simulink model "LQE_x"  (R2022a)
settings: Solver=VariableStepAuto  StartTime=0.0  StopTime=10.0  MaxStep=0.001  RelTol=1e-3
undefined symbols (not defined in the file): A, B, C, K, L
settings Model: Creator=USER  LastModifiedBy=Family
settings SolverCC: AlgebraicLoopSolver=TrustRegion
settings DebuggingCC: UnconnectedInputMsg=warning  UnconnectedOutputMsg=warning  UnconnectedLineMsg=warning  SFMachineParentedDataDiag=warning
settings RTWCC: DLArmComputeVersion=19.05

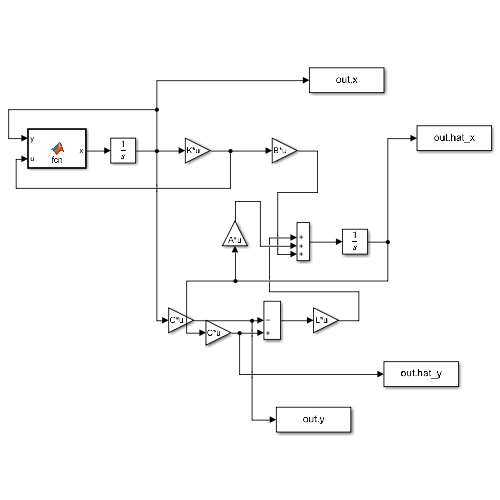
[thumbnail: Simulink's stored preview of the top-level diagram]
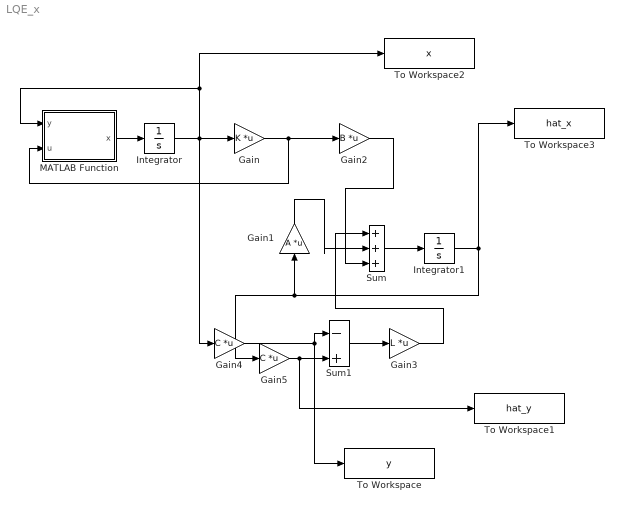
== system LQE_x ==
  Gain : Gain  Gain=K  Multiplication=Matrix(K*u)
  Gain1 : Gain  Gain=A  Multiplication=Matrix(K*u)
  Gain2 : Gain  Gain=B  Multiplication=Matrix(K*u)
  Gain3 : Gain  Gain=L  Multiplication=Matrix(K*u)
  Gain4 : Gain  Gain=C  Multiplication=Matrix(K*u)
  Gain5 : Gain  Gain=C  Multiplication=Matrix(K*u)
  Integrator : Integrator  InitialCondition=[1;0;0.01;0;0.02;0]
  Integrator1 : Integrator  InitialCondition=[0;0.01;0.01;0;0;0]
  MATLAB Function : MATLAB Function  TreatAsAtomicUnit=on
  Sum : Sum  Inputs=|+++
  Sum1 : Sum  Inputs=|-+
  To Workspace : ToWorkspace  VariableName=y  SaveFormat=Timeseries  SampleTime=-1
  To Workspace1 : ToWorkspace  VariableName=hat_y  SaveFormat=Timeseries  SampleTime=-1
  To Workspace2 : ToWorkspace  VariableName=x  SaveFormat=Timeseries  SampleTime=-1
  To Workspace3 : ToWorkspace  VariableName=hat_x  SaveFormat=Timeseries  SampleTime=-1
  wires:
  MATLAB Function/1(x) -> Integrator/1
  Gain/1 -> Gain2/1, MATLAB Function/2(u)
  Integrator/1 -> Gain4/1, Gain/1, To Workspace2/1, MATLAB Function/1(y)
  Gain2/1 -> Sum/3
  Sum/1 -> Integrator1/1
  Integrator1/1 -> To Workspace3/1, Gain1/1, Gain5/1
  Gain1/1 -> Sum/2
  Sum1/1 -> Gain3/1
  Gain4/1 -> To Workspace/1, Sum1/1
  Gain5/1 -> To Workspace1/1, Sum1/2
  Gain3/1 -> Sum/1

== matlab function LQE_x/MATLAB Function ==
  data: y input; u input; x output
function x = fcn(y, u)
    M = 10; %масса тележки
    m1 = 1; %масса маятника 1
    m2 = 2; %масса маятника 2
    l1 = 2; %длина маятника 1
    l2 = 1; %длина маятника 2
    g = 10; %ускорение свпад
    dxdt = zeros(6,1);   
    dxdt(1) = y(2);
    dxdt(2) = -l1*m1*sin(y(3))*(y(5))^2/( M + m1*sin(y(3))^2 + m2*sin(y(4))^2 ) + m1*cos(y(3))*g*sin(y(3))/( M + m1*sin(y(3))^2 + m2*sin(y(4))^2 ) + l2*m2*sin(y(4))*(y(6))^2/( M + m1*sin(y(3))^2 + m2*sin(y(4))^2 ) - m2*cos(y(4))*g*sin(y(4))/( M + m1*sin(y(3))^2 + m2*sin(y(4))^2 ) + u/( M + m1*sin(y(3))^2 + m2*sin(y(4))^2);
    dxdt(3) = y(5);
    dxdt(4) = y(6);
    dxdt(5) = -l1*m1*sin(y(3))*cos(y(3))*(y(5))^2/ (l1* (M + m1*sin(y(3))^2 + m2*sin(y(4))^2)) + g*sin(y(3))*(M+m1+m2*sin(y(4))^2)/ (l1* (M + m1*sin(y(3))^2 + m2*sin(y(4))^2)) + l2*m2*cos(y(3))*sin(y(4))*(y(6))^2/ (l1* (M + m1*sin(y(3))^2 + m2*sin(y(4))^2)) - m2*g*cos(y(3))*cos(y(4))*sin(y(4))/ (l1* (M + m1*sin(y(3))^2 + m2*sin(y(4))^2)) + cos(y(3))*u/ (l1* (M + m1*sin(y(3))^2 + m2*sin(y(4))^2));
    dxdt(6) = l1*m1*sin(y(3))*cos(y(4))*(y(5))^2/ (l2* (M + m1*sin(y(3))^2 + m2*sin(y(4))^2)) - m1*g*cos(y(3))*sin(y(3))*cos(y(4))/ (l2* (M + m1*sin(y(3))^2 + m2*sin(y(4))^2)) - l2*m2*cos(y(4))*sin(y(4))*(y(6))^2/ (l2* (M + m1*sin(y(3))^2 + m2*sin(y(4))^2)) + g*sin(y(4))*(M+m1*sin(y(3))^2+m2)/ (l2* (M + m1*sin(y(3))^2 + m2*sin(y(4))^2)) - cos(y(4))*u/ (l2* (M + m1*sin(y(3))^2 + m2*sin(y(4))^2));
    x = dxdt;
 end
